simulink model "term_block_diagram"  (R2020a)
settings: Solver=VariableStepAuto  StartTime=0.0  StopTime=10.0  RelTol=1e-3
undefined symbols (not defined in the file): Kdi, Kdo, Kpi, Kpo, Kstic, L_grav, theta_off, Ti, Ts, x_ref
settings Model: Creator=Nick  LastModifiedBy=Nick

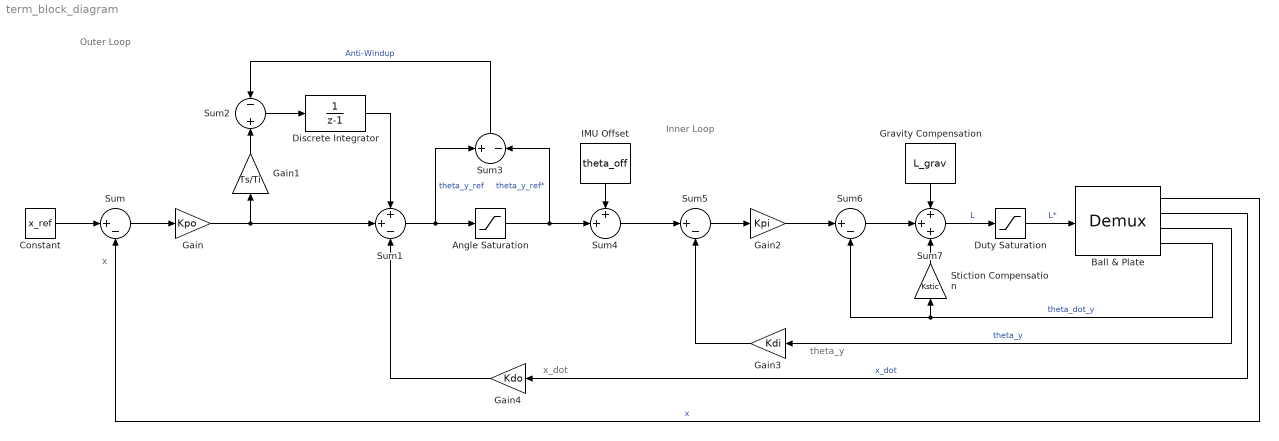
== system term_block_diagram ==
  note: Outer Loop
  note: x
  note: theta_y
  note: x_dot
  note: Inner Loop
  Angle Saturation : Saturate  UpperLimit=12  LowerLimit=-12
  Ball & Plate : Demux
  Constant : Constant  Value=x_ref
  Discrete Integrator : DiscreteTransferFcn  Denominator=[1 -1]
  Duty Saturation : Saturate  UpperLimit=12  LowerLimit=-12
  Gain : Gain  Gain=Kpo
  Gain1 : Gain  Gain=Ts/Ti
  Gain2 : Gain  Gain=Kpi
  Gain3 : Gain  Gain=Kdi
  Gain4 : Gain  Gain=Kdo
  Gravity Compensation : Constant  Value=L_grav
  IMU Offset : Constant  Value=theta_off
  Stiction Compensation : Gain  Gain=Kstic
  Sum : Sum  Inputs=|+-
  Sum1 : Sum  Inputs=++-
  Sum2 : Sum  Inputs=-|+
  Sum3 : Sum  Inputs=+|-
  Sum4 : Sum  Inputs=++|
  Sum5 : Sum  Inputs=|+-
  Sum6 : Sum  Inputs=|+-
  Sum7 : Sum  Inputs=+++
  wires:
  Sum/1 -> Gain/1
  Discrete Integrator/1 -> Sum1/1
  Gain/1 -> Gain1/1, Sum1/2
  Gain1/1 -> Sum2/2
  Sum2/1 -> Discrete Integrator/1
  Constant/1 -> Sum/1
  Sum1/1 -> Sum3/1, Angle Saturation/1  "theta_y_ref"
  Sum3/1 -> Sum2/1  "Anti-Windup"
  Angle Saturation/1 -> Sum3/2, Sum4/2  "theta_y_ref*"
  Sum4/1 -> Sum5/1
  IMU Offset/1 -> Sum4/1
  Gravity Compensation/1 -> Sum7/1
  Gain2/1 -> Sum6/1
  Sum5/1 -> Gain2/1
  Sum6/1 -> Sum7/2
  Sum7/1 -> Duty Saturation/1  "L"
  Ball & Plate/4 -> Stiction Compensation/1, Sum6/2  "theta_dot_y"
  Duty Saturation/1 -> Ball & Plate/1  "L*"
  Ball & Plate/3 -> Gain3/1  "theta_y"
  Gain3/1 -> Sum5/2
  Ball & Plate/2 -> Gain4/1  "x_dot"
  Gain4/1 -> Sum1/3
  Ball & Plate/1 -> Sum/2  "x"
  Stiction Compensation/1 -> Sum7/3
